simulink model "modelo2_fs_step"  (Simulink 7.9)
settings: Solver=ode4  StartTime=0.0  StopTime=t_final  FixedStep=t_step  RelTol=1e-3
InitFcn:
  | modelo2Initialization
undefined symbols (not defined in the file or in its folder): Earth, WGS84
libraries: simulink_extras x2, aerolibfltsims x2, aerolibtransform2 x1, aerolibanimutils x1
settings Model: Creator=claus  LastModifiedBy=claus  SimulationMode=accelerator
settings SolverCC: ShapePreserveControl=EnableAll
settings OptimizationCC: EfficientMapNaN2IntZero=off  SimCompilerOptimization=On  AccelVerboseBuild=on
settings HardwareCC: TargetBitPerLong=64  TargetBitPerPointer=64  TargetIntDivRoundTo=Zero  TargetEndianess=LittleEndian  TargetWordSize=64  TargetHWDeviceType=MATLAB Host  ProdEqTarget=off
settings ModelReferenceCC: EnableParallelModelReferenceBuilds=on
settings CodeAppCC: MaxIdLength=128
settings GRTTargetCC: CombineOutputUpdateFcns=off  GRTInterface=on

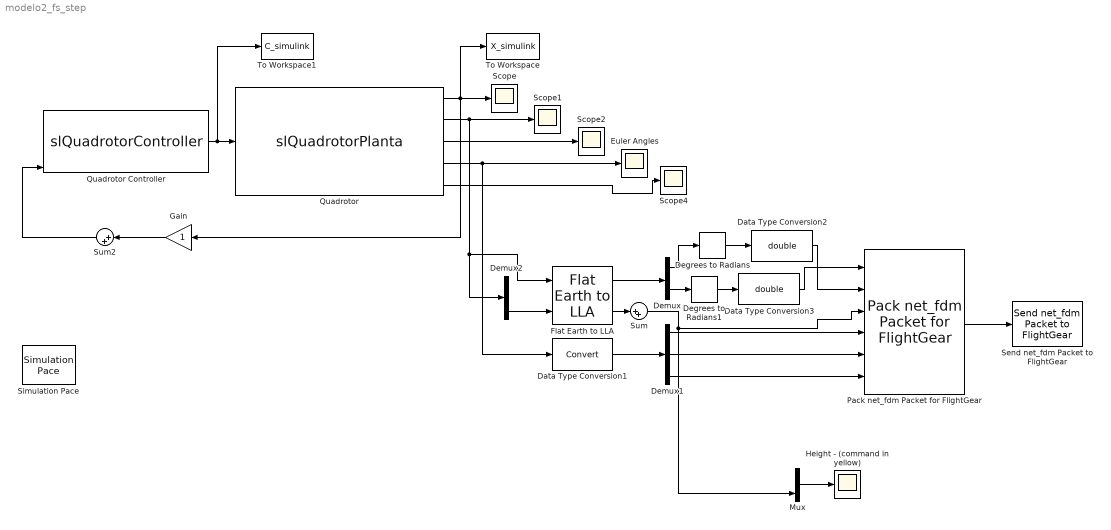
== system modelo2_fs_step ==
  Data Type Conversion1 : DataTypeConversion
  Data Type Conversion2 : DataTypeConversion  OutDataTypeStr=double
  Data Type Conversion3 : DataTypeConversion  OutDataTypeStr=double
  Degrees to Radians : simulink_extras/Transformations/Degrees to Radians
  Degrees to Radians1 : simulink_extras/Transformations/Degrees to Radians
  Demux : Demux  Outputs=2
  Demux1 : Demux  Outputs=3
  Demux2 : Demux  Outputs=3
  Euler Angles : Scope
      settings: TimeRange=20  YMin=-0.25  YMax=3.25  SaveName=ScopeData3
  Flat Earth to LLA : aerolibtransform2/Flat Earth to LLA  units=Metric (MKS)  ptype=Earth (WGS84)  F=1/298.257223563  R=6378137  LL0=[37.6270 -122.3801]  psi=0
  Gain : Gain
  Height - (command in yellow) : Scope
      settings: TimeRange=20  YMin=2.5  YMax=47.5  SaveName=ScopeData6
  Mux : Mux  Inputs=2
  Pack net_fdm Packet for FlightGear : aerolibfltsims/Pack net_fdm Packet for FlightGear  FlightGearVersion=v2.0  ShowPositionAttitudeInputs=on  ShowVelocityAccelerationInputs=off  ShowControlSurfacePositionInputs=off  ShowEngineFuelInputs=off  ShowLandingGearInputs=off  ShowEnvironmentInputs=off  SampleTime=-1
  Quadrotor : M-S-Function  FunctionName=slQuadrotorPlanta
      mask init:
      | slQuadrotorPlantaInitialization
      mask Display:
      | port_label('output', 1, 'state x(1:12)')
      | port_label('output', 2, 'pos (I)')
      | port_label('output', 3, 'vel (B)')
      | port_label('output', 4, 'Euler (I) [Roll Pitch Yaw]')
      | port_label('output', 5, '\omega (B)')
      | port_label('input', 1, 'Control [f1 f2 f3 f4]')
  Quadrotor Controller : M-S-Function  FunctionName=slQuadrotorController
      mask Display:
      | port_label('output', 1, 'Control=[f1 f2 f3 f4]')
      | port_label('input', 1, 'Joystick roll')
      | port_label('input', 2, 'Joystick pitch')
      | port_label('input', 3, 'Joystick yaw')
      | port_label('input', 4, 'Joystick throttle')
      | port_label('input', 5, 'state x(1:12)')
  Scope{,1..2,4} (4 alike) : Scope
      Scope settings: TimeRange=1  YMin=-45  YMax=2.5
      Scope1 settings: TimeRange=20  YMin=-7.5  YMax=22.5
      Scope2 settings: TimeRange=1  YMin=-45  YMax=2.5  SaveName=ScopeData2
      Scope4 settings: TimeRange=1  YMin=-0.01  YMax=0.11  SaveName=ScopeData4
  Send net_fdm Packet to FlightGear : aerolibfltsims/Send net_fdm Packet to FlightGear  DestinationIpAddress=127.0.0.1  DestinationPort=5502  LocalIpPort=-1  varLen=off  SampleTime=-1
  Simulation Pace : aerolibanimutils/Simulation Pace  SimulationPace=1  SleepMode=MATLAB Thread  OutputPaceError=off  SampleTime=0.1
      settings: AttributesFormatString=%<SimulationPace> sec/sec
  Sum : Sum  Inputs=|++
  Sum2 : Sum  Inputs=|++
  To Workspace : ToWorkspace  VariableName=X_simulink  SampleTime=-1  SaveFormat=Timeseries
  To Workspace1 : ToWorkspace  VariableName=C_simulink  SampleTime=-1  SaveFormat=Timeseries
  wires:
  Quadrotor Controller/1 -> Quadrotor/1, To Workspace1/1
  Quadrotor/1 -> Scope/1, To Workspace/1, Gain/1
  Quadrotor/2 -> Demux2/1, Flat Earth to LLA/1, Scope1/1
  Quadrotor/3 -> Scope2/1
  Quadrotor/4 -> Data Type Conversion1/1, Euler Angles/1
  Quadrotor/5 -> Scope4/1
  Pack net_fdm Packet for FlightGear/1 -> Send net_fdm Packet to FlightGear/1
  Demux1/1 -> Pack net_fdm Packet for FlightGear/4
  Demux1/2 -> Pack net_fdm Packet for FlightGear/5
  Demux1/3 -> Pack net_fdm Packet for FlightGear/6
  Data Type Conversion1/1 -> Demux1/1
  Flat Earth to LLA/1 -> Demux/1
  Demux2/3 -> Flat Earth to LLA/2
  Degrees to Radians/1 -> Data Type Conversion2/1
  Degrees to Radians1/1 -> Data Type Conversion3/1
  Demux/1 -> Degrees to Radians/1
  Demux/2 -> Degrees to Radians1/1
  Data Type Conversion3/1 -> Pack net_fdm Packet for FlightGear/1
  Data Type Conversion2/1 -> Pack net_fdm Packet for FlightGear/2
  Flat Earth to LLA/2 -> Sum/1
  Sum/1 -> Pack net_fdm Packet for FlightGear/3, Mux/2
  Mux/1 -> Height - (command in yellow)/1
  Sum2/1 -> Quadrotor Controller/5
  Gain/1 -> Sum2/1
